simulink model "simulink_problem_2"  (R2022b)
settings: Solver=VariableStepAuto  StartTime=0.0  StopTime=10.0  RelTol=1e-3
PreLoadFcn:
  | init;
values from neighbouring files (symbols this model uses):
  J_ew = 1    [init.m]
  s = sind(d)    [graifx.m]    (also in init.m = 1; qube.m = qstate('types'))
  s_max = 2    [init.m]
  T_l = 1    [init.m]
  T_max = 200    [init.m]
  w_s = 1    [init.m]
settings Model: Creator=Administrator  LastModifiedBy=Administrator

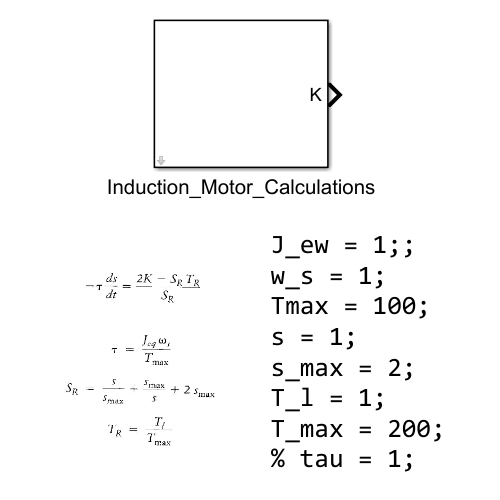
[thumbnail: Simulink's stored preview of the top-level diagram]
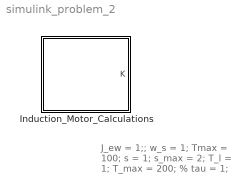
== system simulink_problem_2 ==
  note: J_ew = 1;;
      | w_s = 1;
      | Tmax = 100;
      | s = 1;
      | s_max = 2;
      | T_l = 1;
      | T_max = 200;
      | % tau = 1;
  Induction_Motor_Calculations : Subsystem  mask{J_ew=J_ew, w_s=w_s, T_max=T_max, s=s, s_max=s_max, T_l=T_l}
      mask prompts: J_ew "Inertia:"; w_s "Speed in rad/s:"; T_max "Max Torqwe in N/m:"; s "Speed in rpm:"; s_max "Max speed in rpm:"; T_l "Load Torque in N/m:"
      mask DialogControl Control1 Prompt: Enter parameters below:

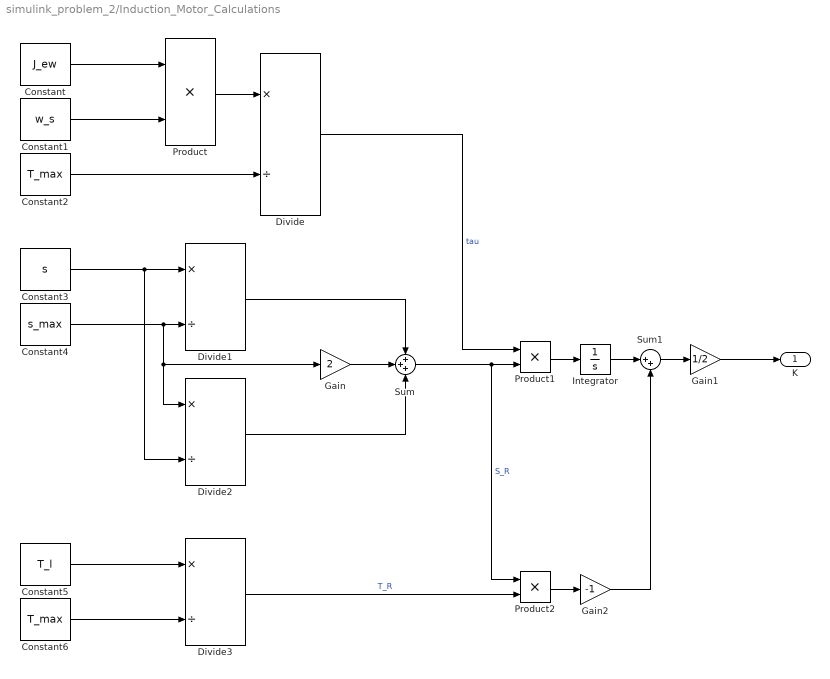
== system simulink_problem_2/Induction_Motor_Calculations ==
  Constant : Constant  Value=J_ew
  Constant1 : Constant  Value=w_s
  Constant2 : Constant  Value=T_max
  Constant3 : Constant  Value=s
  Constant4 : Constant  Value=s_max
  Constant5 : Constant  Value=T_l
  Constant6 : Constant  Value=T_max
  Divide{,1..3} (4 alike) : Product  Inputs=*/
  Gain : Gain  Gain=2
  Gain1 : Gain  Gain=1/2
  Gain2 : Gain  Gain=-1
  Integrator : Integrator
  Product : Product
  Product1 : Product
  Product2 : Product
  Sum : Sum  Inputs=+++
  Sum1 : Sum  Inputs=|++
  K : Outport
  wires:
  Constant5/1 -> Divide3/1
  Constant4/1 -> Gain/1, Divide2/1, Divide1/2
  Constant2/1 -> Divide/2
  Constant3/1 -> Divide2/2, Divide1/1
  Product/1 -> Divide/1
  Divide/1 -> Product1/1  "tau"
  Sum1/1 -> Gain1/1
  Sum/1 -> Product2/1, Product1/2  "S_R"
  Divide1/1 -> Sum/1
  Constant6/1 -> Divide3/2
  Constant/1 -> Product/1
  Product1/1 -> Integrator/1
  Gain/1 -> Sum/2
  Divide2/1 -> Sum/3
  Product2/1 -> Gain2/1
  Constant1/1 -> Product/2
  Integrator/1 -> Sum1/1
  Gain1/1 -> K/1
  Divide3/1 -> Product2/2  "T_R"
  Gain2/1 -> Sum1/2
